simulink model "ODE_reaction_Simulink"  (R2023a)
settings: Solver=FixedStepAuto  StartTime=0.0  StopTime=4.0  FixedStep=0.01  RelTol=1e-3
values from neighbouring files (symbols this model uses):
  C0 = 0    [ODE_reaction_Generator.m]
  Cin = 1    [ODE_reaction_Generator.m]
  Ke = 1    [ODE_reaction_Generator.m]
  tau = 1    [ODE_reaction_Generator.m]
settings Model: Creator=pierr  LastModifiedBy=pierr

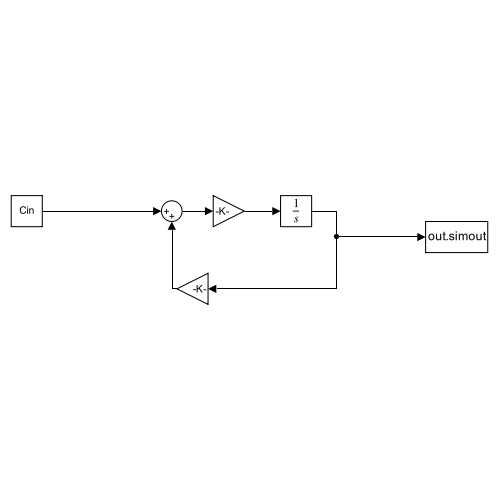
[thumbnail: Simulink's stored preview of the top-level diagram]
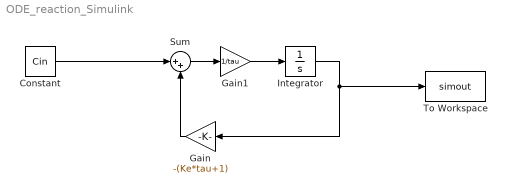
== system ODE_reaction_Simulink ==
  Constant : Constant  Value=Cin
  Gain : Gain  Gain=-(Ke*tau+1)
  Gain1 : Gain  Gain=1/tau
  Integrator : Integrator  InitialCondition=C0
  Sum : Sum  Inputs=|++
  To Workspace : ToWorkspace  VariableName=simout  SaveFormat=Timeseries  SampleTime=-1
  wires:
  Sum/1 -> Gain1/1
  Integrator/1 -> Gain/1, To Workspace/1
  Constant/1 -> Sum/1
  Gain1/1 -> Integrator/1
  Gain/1 -> Sum/2
